simulink subsystem "thermal"  (R2023b)
settings: Solver=VariableStepAuto  StartTime=0.0  StopTime=10.0  RelTol=1e-3
settings Model: Creator=gio  LastModifiedBy=gio

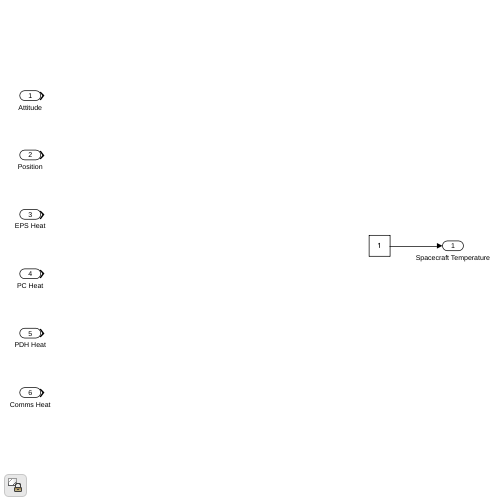
[thumbnail: Simulink's stored preview of the top-level diagram]
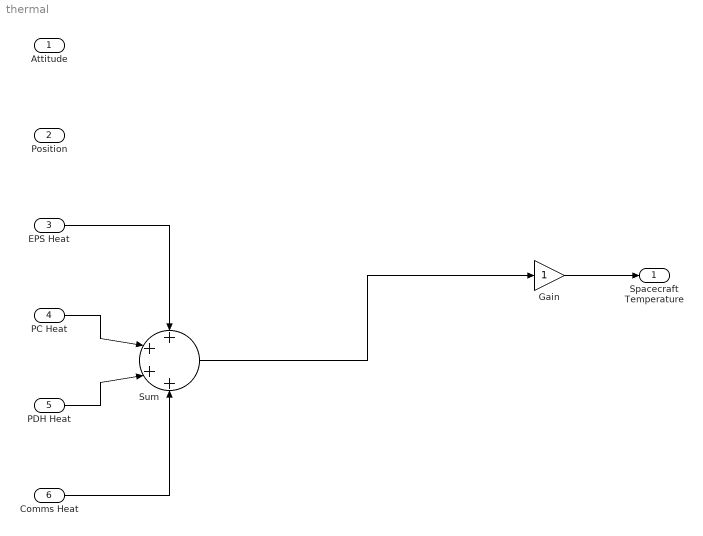
== system thermal ==
  Attitude : Inport
  Position : Inport  Port=2
  EPS Heat : Inport  Port=3
  PC Heat : Inport  Port=4
  PDH Heat : Inport  Port=5
  Comms Heat : Inport  Port=6
  Gain : Gain
  Sum : Sum  Inputs=++++
  Spacecraft Temperature : Outport
  wires:
  EPS Heat/1 -> Sum/1
  PC Heat/1 -> Sum/2
  PDH Heat/1 -> Sum/3
  Comms Heat/1 -> Sum/4
  Gain/1 -> Spacecraft Temperature/1
  Sum/1 -> Gain/1
